simulink model "PVPanelAnn"  (R2018a)
settings: Solver=FixedStepDiscrete  StartTime=0.0  StopTime=3.0  FixedStep=10e-6  RelTol=1e-3
libraries: neural x37, powerlib x18, simulink x2, re_lib x1, powerlib_meascontrol x1
(part 2 of 2)

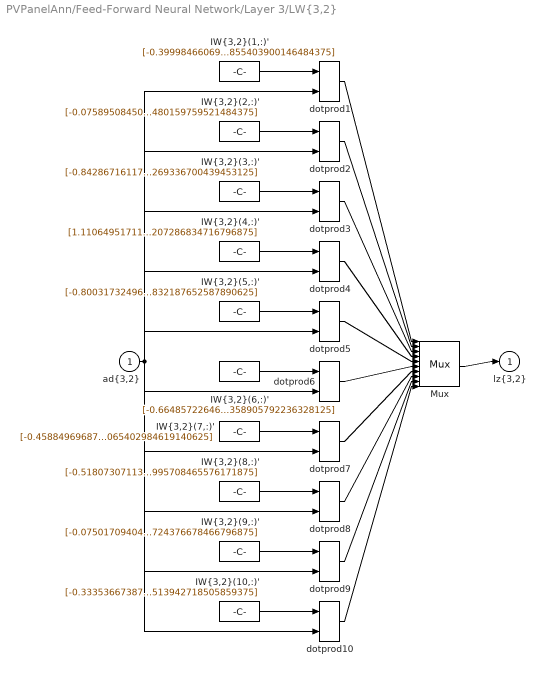
== system PVPanelAnn/Feed-Forward Neural Network/Layer 3/LW{3,2} ==
  "ad{3,2}" : Inport  PortDimensions=10
      mask Display: e = 0.06;c1 = [120 230 180]/255;c2 = ([120 230 180]+0)/(256+128);c3 = ([120 230 180]+128)/(256+128);patch([0 1 1 0],[0 0 1 1],c1);patch([0 1 1 1-e 1-e 0+e],[0 0 1 1-e 0+e 0+e],c2);patch([0 0 1 1-e 0+e 0+e],[0 1 1 1-e 1-e 0+e],c3);plot([0 1 1 0 0],[0 0 1 1 0]);
  "IW{3,2}(1,:)'" : Constant  Value=[-0.3999846606919224001330803730525076389312744140625;0.869918937407937686856485015596263110637664794921875;-0.38301463792397105745379803920513950288295745849609375;-0.89957239528069476985905339461169205605983734130859375;0.278496550774055273702600743490620516240596771240234375;-0.47808471685320619304349065714632160961627960205078125;0.7822134109873974949778130394406616687774658203125;-0.148908453103518689797368779181852005422115325927734375;0.05991901667434547384960552562915836460888385772705078125;0.53693694364701372023773728869855403900146484375]
      mask Display: e = 0.06;c1 = [120 150 230]/255;c2 = ([120 150 230]+0)/383;c3 = ([120 150 230]+128)/383;patch([0 1 1 0],[0 0 1 1],c1);patch([0 1 1 1-e 1-e 0+e],[0 0 1 1-e 0+e 0+e],c2);patch([0 0 1 1-e 0+e 0+e],[0 1 1 1-e 1-e 0+e],c3);plot([0 1 1 0 0],[0 0 1 1 0]);disp('weights');
  "IW{3,2}(10,:)'" : Constant  Value=[-0.3335366738703509081886977583053521811962127685546875;0.8716491908409949029845620316336862742900848388671875;-0.5562354869371726184823501171194948256015777587890625;0.60687793223369645989606624425505287945270538330078125;-0.002823750865846845481410554157264414243400096893310546875;-0.780880359966358295054078553221188485622406005859375;-0.62193568994668113614210369632928632199764251708984375;-0.284832365948058663374098387066624127328395843505859375;0.148392393031686442572691930763539858162403106689453125;0.74796184528993803208862800602219067513942718505859375]
      mask Display: e = 0.06;c1 = [120 150 230]/255;c2 = ([120 150 230]+0)/383;c3 = ([120 150 230]+128)/383;patch([0 1 1 0],[0 0 1 1],c1);patch([0 1 1 1-e 1-e 0+e],[0 0 1 1-e 0+e 0+e],c2);patch([0 0 1 1-e 0+e 0+e],[0 1 1 1-e 1-e 0+e],c3);plot([0 1 1 0 0],[0 0 1 1 0]);disp('weights');
  "IW{3,2}(2,:)'" : Constant  Value=[-0.07589508450538652584160814740243949927389621734619140625;0.9608167461922623164838341836002655327320098876953125;0.33727821283747105862715898183523677289485931396484375;0.2230341467841015223871892203533207066357135772705078125;-0.175479300906613511212839284780784510076045989990234375;-0.434879062001289840022622001924901269376277923583984375;0.82160300201090430416428489479585550725460052490234375;-0.9683139308041806003757301368750631809234619140625;0.410283986710281933785182673091185279190540313720703125;-0.238156656728728266525507706319331191480159759521484375]
      mask Display: e = 0.06;c1 = [120 150 230]/255;c2 = ([120 150 230]+0)/383;c3 = ([120 150 230]+128)/383;patch([0 1 1 0],[0 0 1 1],c1);patch([0 1 1 1-e 1-e 0+e],[0 0 1 1-e 0+e 0+e],c2);patch([0 0 1 1-e 0+e 0+e],[0 1 1 1-e 1-e 0+e],c3);plot([0 1 1 0 0],[0 0 1 1 0]);disp('weights');
  "IW{3,2}(3,:)'" : Constant  Value=[-0.84286716117852311658253938730922527611255645751953125;-0.77943358573383958454172670826665125787258148193359375;0.286533028630781061441012980139930732548236846923828125;0.68868301669111053886496165432617999613285064697265625;-0.447957157397504246443276088029961101710796356201171875;0.31590125548953562617526813482982106506824493408203125;0.57324759215105391962907788183656521141529083251953125;0.092153160764183450481823456357233226299285888671875;-0.0816075094175741921898037389837554655969142913818359375;-0.73447079100634671267044950582203455269336700439453125]
      mask Display: e = 0.06;c1 = [120 150 230]/255;c2 = ([120 150 230]+0)/383;c3 = ([120 150 230]+128)/383;patch([0 1 1 0],[0 0 1 1],c1);patch([0 1 1 1-e 1-e 0+e],[0 0 1 1-e 0+e 0+e],c2);patch([0 0 1 1-e 0+e 0+e],[0 1 1 1-e 1-e 0+e],c3);plot([0 1 1 0 0],[0 0 1 1 0]);disp('weights');
  "IW{3,2}(4,:)'" : Constant  Value=[1.110649517118452056507749148295260965824127197265625;0.5459382548380329325254933792166411876678466796875;0.07669214459164029606963453034040867350995540618896484375;0.393147241269902192328800083487294614315032958984375;-0.1393901081632832605894378730226890183985233306884765625;-0.511297288515500714112249625031836330890655517578125;-0.53751111068689716443458337380434386432170867919921875;-0.07537531899354450726224996515156817622482776641845703125;0.74113759021102254553881039100815542042255401611328125;-0.541418381602891685133727150969207286834716796875]
      mask Display: e = 0.06;c1 = [120 150 230]/255;c2 = ([120 150 230]+0)/383;c3 = ([120 150 230]+128)/383;patch([0 1 1 0],[0 0 1 1],c1);patch([0 1 1 1-e 1-e 0+e],[0 0 1 1-e 0+e 0+e],c2);patch([0 0 1 1-e 0+e 0+e],[0 1 1 1-e 1-e 0+e],c3);plot([0 1 1 0 0],[0 0 1 1 0]);disp('weights');
  "IW{3,2}(5,:)'" : Constant  Value=[-0.800317324961350440304386211209930479526519775390625;-0.487994804901162648747003913740627467632293701171875;0.472520543861635167193213646896765567362308502197265625;-0.747237069818296628653797597507946193218231201171875;-0.08499634211297439623233884731234866194427013397216796875;0.639966007929543057031196440220810472965240478515625;0.19340712680851990246111427040887065231800079345703125;0.511428081714864202211856536450795829296112060546875;0.40887026642136603538091321752290241420269012451171875;-0.74685944436614060126800040961825288832187652587890625]
      mask Display: e = 0.06;c1 = [120 150 230]/255;c2 = ([120 150 230]+0)/383;c3 = ([120 150 230]+128)/383;patch([0 1 1 0],[0 0 1 1],c1);patch([0 1 1 1-e 1-e 0+e],[0 0 1 1-e 0+e 0+e],c2);patch([0 0 1 1-e 0+e 0+e],[0 1 1 1-e 1-e 0+e],c3);plot([0 1 1 0 0],[0 0 1 1 0]);disp('weights');
  "IW{3,2}(6,:)'" : Constant  Value=[-0.66485722646626388421253750493633560836315155029296875;-0.04060210922424743740233310518306097947061061859130859375;0.16375058962347777136159265864989720284938812255859375;-0.1916306965280981933208437339999363757669925689697265625;-0.51468487503972648600125694429152645170688629150390625;0.9356067642331691303070329013280570507049560546875;-0.75673626426666296129752709020976908504962921142578125;0.129277668629173059233750109342508949339389801025390625;0.920881661753318869756412823335267603397369384765625;-0.312192067577979515125008447284926660358905792236328125]
      mask Display: e = 0.06;c1 = [120 150 230]/255;c2 = ([120 150 230]+0)/383;c3 = ([120 150 230]+128)/383;patch([0 1 1 0],[0 0 1 1],c1);patch([0 1 1 1-e 1-e 0+e],[0 0 1 1-e 0+e 0+e],c2);patch([0 0 1 1-e 0+e 0+e],[0 1 1 1-e 1-e 0+e],c3);plot([0 1 1 0 0],[0 0 1 1 0]);disp('weights');
  "IW{3,2}(7,:)'" : Constant  Value=[-0.458849696871556744781628367491066455841064453125;0.1775032042689372036026185242008068598806858062744140625;-1.2224105045717863493592858503689058125019073486328125;-0.1341662349867452641571929916608496569097042083740234375;0.304638395586930565972494378002011217176914215087890625;0.83125539407307857953099983205902390182018280029296875;-0.303320512860833446655561829174985177814960479736328125;0.57385802331292101730042531926301307976245880126953125;0.1071738724870948955558702664347947575151920318603515625;-0.267066801926624963758882813635864295065402984619140625]
      mask Display: e = 0.06;c1 = [120 150 230]/255;c2 = ([120 150 230]+0)/383;c3 = ([120 150 230]+128)/383;patch([0 1 1 0],[0 0 1 1],c1);patch([0 1 1 1-e 1-e 0+e],[0 0 1 1-e 0+e 0+e],c2);patch([0 0 1 1-e 0+e 0+e],[0 1 1 1-e 1-e 0+e],c3);plot([0 1 1 0 0],[0 0 1 1 0]);disp('weights');
  "IW{3,2}(8,:)'" : Constant  Value=[-0.51807307113571232637383445762679912149906158447265625;0.7609322707975600952323702585999853909015655517578125;-0.6525205075667031007213836346636526286602020263671875;0.8364000484267222201850700002978555858135223388671875;-0.4473999293771646623696369715617038309574127197265625;-0.2369518394958663176641522341014933772385120391845703125;-0.301751757875491743998708216167869977653026580810546875;-0.82229388056661145700587667306535877287387847900390625;-0.281605979875654721666933255619369447231292724609375;0.0366475257773832552299353437774698249995708465576171875]
      mask Display: e = 0.06;c1 = [120 150 230]/255;c2 = ([120 150 230]+0)/383;c3 = ([120 150 230]+128)/383;patch([0 1 1 0],[0 0 1 1],c1);patch([0 1 1 1-e 1-e 0+e],[0 0 1 1-e 0+e 0+e],c2);patch([0 0 1 1-e 0+e 0+e],[0 1 1 1-e 1-e 0+e],c3);plot([0 1 1 0 0],[0 0 1 1 0]);disp('weights');
  "IW{3,2}(9,:)'" : Constant  Value=[-0.07501709404785657231418127821598318405449390411376953125;-0.1640989556511952829342959603309282101690769195556640625;0.9802271502012300796735644325963221490383148193359375;-0.69083573545794607628778294383664615452289581298828125;-0.08556944467633280371199333558251964859664440155029296875;0.3080324207150397786136863942374475300312042236328125;-0.5680891706315167599683491062023676931858062744140625;-0.9398749221788553764866946949041448533535003662109375;-0.64359087421890437408222851445316337049007415771484375;-0.060660847433809166051599248703496414236724376678466796875]
      mask Display: e = 0.06;c1 = [120 150 230]/255;c2 = ([120 150 230]+0)/383;c3 = ([120 150 230]+128)/383;patch([0 1 1 0],[0 0 1 1],c1);patch([0 1 1 1-e 1-e 0+e],[0 0 1 1-e 0+e 0+e],c2);patch([0 0 1 1-e 0+e 0+e],[0 1 1 1-e 1-e 0+e],c3);plot([0 1 1 0 0],[0 0 1 1 0]);disp('weights');
  Mux : Mux  Inputs=10
      mask Display: e = 0.06;c1 = [120 150 230]/255;c2 = ([120 150 230]+0)/383;c3 = ([120 150 230]+128)/383;patch([0 1 1 0],[0 0 1 1],c1);patch([0 1 1 1-e 1-e 0+e],[0 0 1 1-e 0+e 0+e],c2);patch([0 0 1 1-e 0+e 0+e],[0 1 1 1-e 1-e 0+e],c3);plot([0 1 1 0 0],[0 0 1 1 0]);disp('Mux');
  dotprod{1..10} (10 alike) : neural/Weight Functions/dotprod
  "lz{3,2}" : Outport
      mask Display: e = 0.06;c1 = [120 230 180]/255;c2 = ([120 230 180]+0)/(256+128);c3 = ([120 230 180]+128)/(256+128);patch([0 1 1 0],[0 0 1 1],c1);patch([0 1 1 1-e 1-e 0+e],[0 0 1 1-e 0+e 0+e],c2);patch([0 0 1 1-e 0+e 0+e],[0 1 1 1-e 1-e 0+e],c3);plot([0 1 1 0 0],[0 0 1 1 0]);
  wires:
  "IW{3,2}(1,:)'"/1 -> dotprod1/1
  "ad{3,2}"/1 -> dotprod1/2, dotprod2/2, dotprod3/2, dotprod4/2, dotprod5/2, dotprod6/2, dotprod7/2, dotprod8/2, dotprod9/2, dotprod10/2
  dotprod1/1 -> Mux/1
  "IW{3,2}(2,:)'"/1 -> dotprod2/1
  dotprod2/1 -> Mux/2
  "IW{3,2}(3,:)'"/1 -> dotprod3/1
  dotprod3/1 -> Mux/3
  "IW{3,2}(4,:)'"/1 -> dotprod4/1
  dotprod4/1 -> Mux/4
  "IW{3,2}(5,:)'"/1 -> dotprod5/1
  dotprod5/1 -> Mux/5
  "IW{3,2}(6,:)'"/1 -> dotprod6/1
  dotprod6/1 -> Mux/6
  "IW{3,2}(7,:)'"/1 -> dotprod7/1
  dotprod7/1 -> Mux/7
  "IW{3,2}(8,:)'"/1 -> dotprod8/1
  dotprod8/1 -> Mux/8
  "IW{3,2}(9,:)'"/1 -> dotprod9/1
  dotprod9/1 -> Mux/9
  "IW{3,2}(10,:)'"/1 -> dotprod10/1
  dotprod10/1 -> Mux/10
  Mux/1 -> "lz{3,2}"/1

== system PVPanelAnn/Feed-Forward Neural Network/Layer 4/Delays 1 ==
  "p{4}" : Inport  PortDimensions=10
      mask Display: e = 0.06;c1 = [120 230 180]/255;c2 = ([120 230 180]+0)/(256+128);c3 = ([120 230 180]+128)/(256+128);patch([0 1 1 0],[0 0 1 1],c1);patch([0 1 1 1-e 1-e 0+e],[0 0 1 1-e 0+e 0+e],c2);patch([0 0 1 1-e 0+e 0+e],[0 1 1 1-e 1-e 0+e],c3);plot([0 1 1 0 0],[0 0 1 1 0]);
  mux : Mux  Inputs=1
      mask Display: e = 0.06;c1 = [120 150 230]/255;c2 = ([120 150 230]+0)/383;c3 = ([120 150 230]+128)/383;patch([0 1 1 0],[0 0 1 1],c1);patch([0 1 1 1-e 1-e 0+e],[0 0 1 1-e 0+e 0+e],c2);patch([0 0 1 1-e 0+e 0+e],[0 1 1 1-e 1-e 0+e],c3);plot([0 1 1 0 0],[0 0 1 1 0]);disp('Mux')
  "pd{4,3}" : Outport
      mask Display: e = 0.06;c1 = [120 230 180]/255;c2 = ([120 230 180]+0)/(256+128);c3 = ([120 230 180]+128)/(256+128);patch([0 1 1 0],[0 0 1 1],c1);patch([0 1 1 1-e 1-e 0+e],[0 0 1 1-e 0+e 0+e],c2);patch([0 0 1 1-e 0+e 0+e],[0 1 1 1-e 1-e 0+e],c3);plot([0 1 1 0 0],[0 0 1 1 0]);
  wires:
  "p{4}"/1 -> mux/1
  mux/1 -> "pd{4,3}"/1

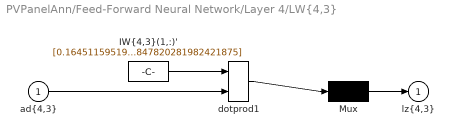
== system PVPanelAnn/Feed-Forward Neural Network/Layer 4/LW{4,3} ==
  "ad{4,3}" : Inport  PortDimensions=10
      mask Display: e = 0.06;c1 = [120 230 180]/255;c2 = ([120 230 180]+0)/(256+128);c3 = ([120 230 180]+128)/(256+128);patch([0 1 1 0],[0 0 1 1],c1);patch([0 1 1 1-e 1-e 0+e],[0 0 1 1-e 0+e 0+e],c2);patch([0 0 1 1-e 0+e 0+e],[0 1 1 1-e 1-e 0+e],c3);plot([0 1 1 0 0],[0 0 1 1 0]);
  "IW{4,3}(1,:)'" : Constant  Value=[0.164511595194792803464878261365811340510845184326171875;1.0502385251391472831272722032736055552959442138671875;0.295280439892644797073018025912460871040821075439453125;0.78025847718473106962022711741155944764614105224609375;-0.26989225242252512515506168710999190807342529296875;0.52784334872508165137361402230453677475452423095703125;0.11383992554494480609061923814806505106389522552490234375;0.1890799656469654699275650955314631573855876922607421875;0.277027197708985484236876573049812577664852142333984375;-1.0217684693126738437740641529671847820281982421875]
      mask Display: e = 0.06;c1 = [120 150 230]/255;c2 = ([120 150 230]+0)/383;c3 = ([120 150 230]+128)/383;patch([0 1 1 0],[0 0 1 1],c1);patch([0 1 1 1-e 1-e 0+e],[0 0 1 1-e 0+e 0+e],c2);patch([0 0 1 1-e 0+e 0+e],[0 1 1 1-e 1-e 0+e],c3);plot([0 1 1 0 0],[0 0 1 1 0]);disp('weights');
  Mux : Mux  Inputs=1
      mask Display: e = 0.06;c1 = [120 150 230]/255;c2 = ([120 150 230]+0)/383;c3 = ([120 150 230]+128)/383;patch([0 1 1 0],[0 0 1 1],c1);patch([0 1 1 1-e 1-e 0+e],[0 0 1 1-e 0+e 0+e],c2);patch([0 0 1 1-e 0+e 0+e],[0 1 1 1-e 1-e 0+e],c3);plot([0 1 1 0 0],[0 0 1 1 0]);disp('Mux');
  dotprod1 : neural/Weight Functions/dotprod
  "lz{4,3}" : Outport
      mask Display: e = 0.06;c1 = [120 230 180]/255;c2 = ([120 230 180]+0)/(256+128);c3 = ([120 230 180]+128)/(256+128);patch([0 1 1 0],[0 0 1 1],c1);patch([0 1 1 1-e 1-e 0+e],[0 0 1 1-e 0+e 0+e],c2);patch([0 0 1 1-e 0+e 0+e],[0 1 1 1-e 1-e 0+e],c3);plot([0 1 1 0 0],[0 0 1 1 0]);
  wires:
  "IW{4,3}(1,:)'"/1 -> dotprod1/1
  "ad{4,3}"/1 -> dotprod1/2
  dotprod1/1 -> Mux/1
  Mux/1 -> "lz{4,3}"/1
